simulink model "CommandEnEffortavecPosition"  (R2020b)
settings: Solver=FixedStepAuto  StartTime=0.0  StopTime=10  RelTol=1e-3
undefined symbols (not defined in the file): B, Beta, kc, ke, ki, Kipos, kp, Kpos, M, w0, wu, x, xd, xo
settings Model: Creator=Laura  LastModifiedBy=Laura

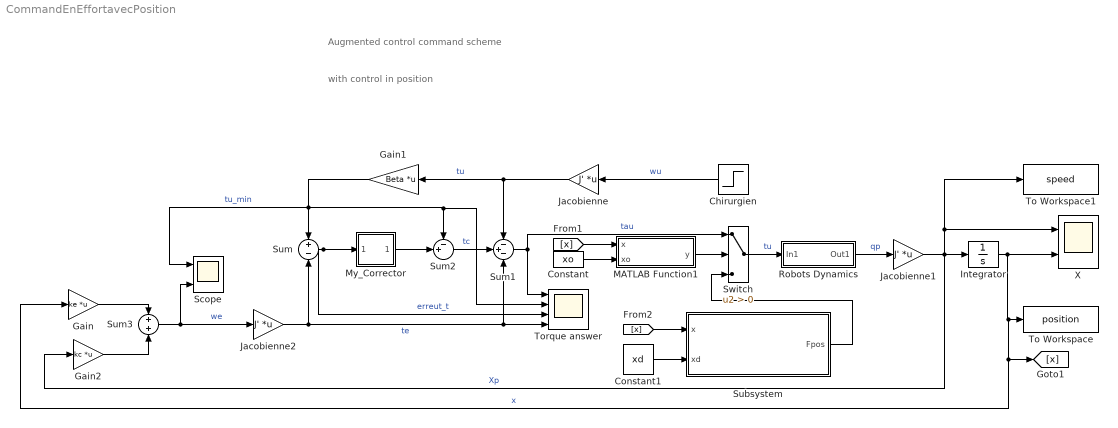
== system CommandEnEffortavecPosition ==
  note: Augmented control command scheme
  note: with control in position
  Chirurgien : Step  Before=w0  After=wu  SampleTime=0  VectorParams1D=off
  Constant : Constant  Value=xo  VectorParams1D=off
  Constant1 : Constant  Value=xd
  Gain : Gain  Gain=ke  Multiplication=Matrix(K*u)
  Gain1 : Gain  Gain=Beta  Multiplication=Matrix(K*u)
  Gain2 : Gain  Gain=kc  Multiplication=Matrix(K*u)
  Integrator : Integrator  InitialCondition=x
  Jacobienne : Gain  Gain=J'  Multiplication=Matrix(K*u)
  Jacobienne1 : Gain  Gain=J'  Multiplication=Matrix(K*u)
  Jacobienne2 : Gain  Gain=J'  Multiplication=Matrix(K*u)
  MATLAB Function1 : MATLAB Function  TreatAsAtomicUnit=on
  My_Corrector : Subsystem
      mask Display: disp('PI')
  Robots Dynamics : Subsystem
      mask Display: disp('(Ms + B)^-1')
  Scope : Scope  NumInputPorts=2
  Subsystem : Subsystem
      mask Display: disp("Position Control")
  Sum : Sum  Inputs=+|-
  Sum1 : Sum  Inputs=-+-
  Sum2 : Sum  Inputs=-+|
  Sum3 : Sum  Inputs=+|+
  Switch : Switch  Criteria=u2 > Threshold
  To Workspace : ToWorkspace  VariableName=position  SampleTime=0.03
  To Workspace1 : ToWorkspace  VariableName=speed  SampleTime=0.03
  Torque answer : Scope  NumInputPorts=4
  X : Scope  NumInputPorts=2
  wires:
  Jacobienne2/1 -> Sum/2, Torque answer/4, Sum1/3  "te"
  Robots Dynamics/1(Out1) -> Jacobienne1/1  "qp"
  Chirurgien/1 -> Jacobienne/1  "wu"
  Jacobienne/1 -> Gain1/1, Sum1/1  "tu"
  Gain1/1 -> Scope/1, Torque answer/2, Sum2/1, Sum/1  "tu_min"
  Sum2/1 -> Sum1/2  "tc"
  Jacobienne1/1 -> To Workspace1/1, X/1, Gain2/1, Integrator/1  "Xp"
  Sum/1 -> My_Corrector/1(erreut_t), Torque answer/3  "erreut_t"
  My_Corrector/1(Out1) -> Sum2/2
  Integrator/1 -> X/2, Gain/1, [x], To Workspace/1  "x"
  Sum1/1 -> Torque answer/1, Switch/1  "tau"
  Gain/1 -> Sum3/1
  Gain2/1 -> Sum3/2
  Sum3/1 -> Scope/2, Jacobienne2/1  "we"
  MATLAB Function1/1(y) -> Switch/2
  Subsystem/1(Fpos) -> Switch/3
  Switch/1 -> Robots Dynamics/1(In1)  "tu"
  Constant/1 -> MATLAB Function1/2(xo)
  [x] -> MATLAB Function1/1(x)
  [x] -> Subsystem/1(x)
  Constant1/1 -> Subsystem/2(xd)

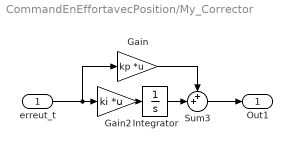
== system CommandEnEffortavecPosition/My_Corrector ==
  erreut_t : Inport
  Gain : Gain  Gain=kp  Multiplication=Matrix(K*u)
  Gain2 : Gain  Gain=ki  Multiplication=Matrix(K*u)
  Integrator : Integrator  InitialCondition=w0
  Sum3 : Sum  Inputs=++|
  Out1 : Outport
  wires:
  Sum3/1 -> Out1/1
  Gain/1 -> Sum3/1
  Gain2/1 -> Integrator/1
  Integrator/1 -> Sum3/2
  erreut_t/1 -> Gain/1, Gain2/1

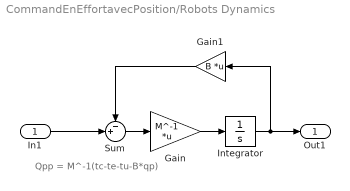
== system CommandEnEffortavecPosition/Robots Dynamics ==
  note: Qpp = M^-1(tc-te-tu-B*qp)
  In1 : Inport
  Gain : Gain  Gain=M^-1  Multiplication=Matrix(K*u)
  Gain1 : Gain  Gain=B  Multiplication=Matrix(K*u)
  Integrator : Integrator
  Sum : Sum  Inputs=-+|
  Out1 : Outport
  wires:
  Gain/1 -> Integrator/1
  Sum/1 -> Gain/1
  Gain1/1 -> Sum/1
  Integrator/1 -> Gain1/1, Out1/1
  In1/1 -> Sum/2

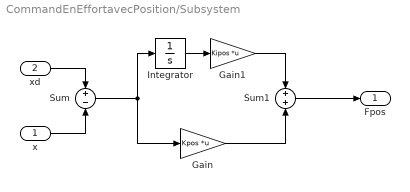
== system CommandEnEffortavecPosition/Subsystem ==
  x : Inport
  xd : Inport  Port=2
  Gain : Gain  Gain=Kpos  Multiplication=Matrix(K*u)
  Gain1 : Gain  Gain=Kipos  Multiplication=Matrix(K*u)
  Integrator : Integrator
  Sum : Sum  Inputs=+|-
  Sum1 : Sum  Inputs=+|+
  Fpos : Outport
  wires:
  x/1 -> Sum/2
  xd/1 -> Sum/1
  Sum/1 -> Gain/1, Integrator/1
  Gain/1 -> Sum1/2
  Integrator/1 -> Gain1/1
  Gain1/1 -> Sum1/1
  Sum1/1 -> Fpos/1

== matlab function CommandEnEffortavecPosition/MATLAB Function1 ==
  data: x input; y output; xo input
function y = isInside(x,xo)
% Function that calculates if the position of the robot is inside of the organ
%x = Robot positio
%xo = Organ Position

ro = 0.15; %rayon d'organe (m)
d = sqrt((xo(1)-x(1))^2 + (xo(2)-x(2))^2);
  
if d <= ro
    y = true;
 else 
    y = false;
end
